simulink model "heating_cooling_process"  (Simulink 3.00)
libraries: mathlib x4, modellib x3, genlib x1

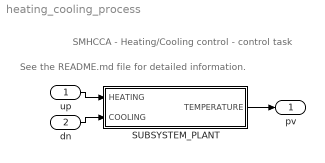
== system heating_cooling_process ==
  note: See the README.md file for detailed information.
  note: SMHCCA - Heating/Cooling control - control task
  up : Inport  Port=1
  dn : Inport  Port=2
  SUBSYSTEM_PLANT : Subsystem
      mask Type: REX sequence
  pv : Outport  Port=1
  wires:
  SUBSYSTEM_PLANT/1(TEMPERATURE) -> pv/1
  dn/1 -> SUBSYSTEM_PLANT/2(COOLING)
  up/1 -> SUBSYSTEM_PLANT/1(HEATING)

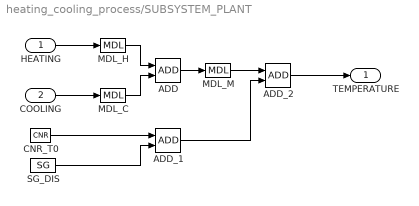
== system heating_cooling_process/SUBSYSTEM_PLANT ==
  HEATING : Inport  Port=1
  COOLING : Inport  Port=2
  ADD : mathlib/ADD
  ADD_1 : mathlib/ADD
  ADD_2 : mathlib/ADD
  CNR_T0 : mathlib/CNR  ycn=20
  MDL_C : modellib/MDL  k0=-1  del=0  tau1=10  tau2=10  nmax=100
  MDL_H : modellib/MDL  k0=1  del=0  tau1=10  tau2=10  nmax=100
  MDL_M : modellib/MDL  k0=500  del=0  tau1=100  tau2=1  nmax=100
  SG_DIS : genlib/SG  isig=1: SINE  amp=0  freq=1  phase=0  ifrunit=1: Hz  iphunit=1: degrees  offset=0
  TEMPERATURE : Outport  Port=1
  wires:
  ADD/1 -> MDL_M/1
  ADD_1/1 -> ADD_2/2
  ADD_2/1 -> TEMPERATURE/1
  CNR_T0/1 -> ADD_1/1
  COOLING/1 -> MDL_C/1
  HEATING/1 -> MDL_H/1
  MDL_C/1 -> ADD/2
  MDL_H/1 -> ADD/1
  MDL_M/1 -> ADD_2/1
  SG_DIS/1 -> ADD_1/2
